simulink model "parent_model_2020a"  (R2020a)
settings: Solver=VariableStepAuto  StartTime=0.0  StopTime=10.0  RelTol=1e-3
libraries: sdl_lib x13, nesl_utility x9, autolibmappedmotor x4, autolibdatasheetbattery x1
settings Model: Creator=True  LastModifiedBy=True

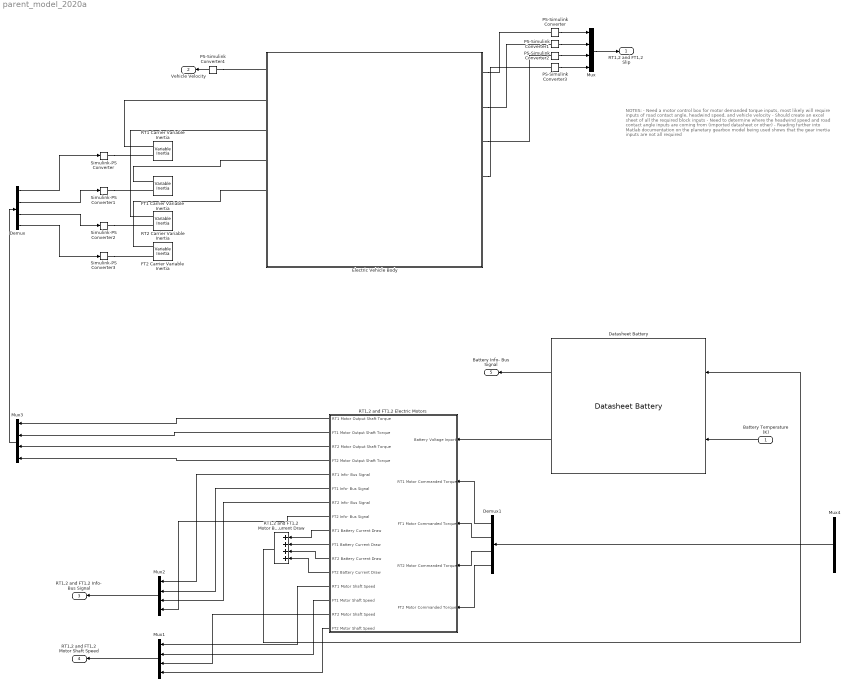
== system parent_model_2020a ==
  note: NOTES:
      | - Need a motor control box for motor demanded torque inputs, most likely will require inputs of road contact angle, headwind speed, and vehicle velocity
      |
      | - Should create an excel sheet of all the required block inputs
      |
      | - Need to determine where the headwind speed and road contact angle inputs are coming from (imported datasheet or other)
      |
      | - Reading further into Matlab documentation on the planetary gearbox model being used shows that the gear inertia inputs are not all required
  Battery Temperature (K) : Inport
  Datasheet Battery : autolibdatasheetbattery/Datasheet Battery  CapacityCtrl=Parameter  OutputVlt=Unfiltered  BattChargeMax=100  Em=[2.8 3.228 3.284 3.361 3.408 3.427 3.472 3.477 3.493 3.504 3.516 3.528 3.537 3.545 3.555 3.561 3.566 3.576 3.587 3.589 3.594 3.6 3.608 3.61 3.616 3.619 3.626 3.632 3.637 3.64 3.645 3.646 3.652 3.655 3.658 3.661 3.664 3.668 3.673 3.678 3.68 3.681 3.686 3.692 3.699 3.702 3.705 3.71 3.717 3.723 3.728 3.733 3.735 3.742 3.749 3.755 3.761 3.768 3.773 3.78 3.791 3.798 3.798 3.814 3.818 3.825 3.841 3.846 3.855 3.863 3.877 3.885 3.894 3.907 3.919 3.926 3.935 3.944 3.954 3.964 3.974 3.988 3.998 4.014 4.029 4.034 4.047 4.065 4.074 4.086 4.097 4.131 4.126 4.138 4.15 4.18 4.174 4.187 4.207 4.231 4.221]  CapLUTBp=[0 0.01 0.02 0.03 0.04 0.05 0.06 0.07 0.08 0.09 0.1 0.11 0.12 0.13 0.14 0.15 0.16 0.17 0.18 0.19 0.2 0.21 0.22 0.23 0.24 0.25 0.26 0.27 0.28 0.29 0.3 0.31 0.32 0.33 0.34 0.35 0.36 0.37 0.38 0.39 0.4 0.41 0.42 0.43 0.44 0.45 0.46 0.47 0.48 0.49 0.5 0.51 0.52 0.53 0.54 0.55 0.56 0.57 0.58 0.59 0.6 0.61 0.62 0.63 0.64 0.65 0.66 0.67 0.68 0.69 0.7 0.71 0.72 0.73 0.74 0.75 0.76 0.77 0.78 0.79 0.8 0.81 0.82 0.83 0.84 0.85 0.86 0.87 0.88 0.89 0.9 0.91 0.92 0.93 0.94 0.95 0.96 0.97 0.98 0.99 1]  RInt=[0.008846 0.009319 0.009027 0.00847 0.01032 0.01314;0.006389 0.006554 0.005553 0.005525 0.006043 0.007805;0.004364 0.004101 0.00406 0.003452 0.003846 0.004517;0.002031 0.002563 0.002532 0.00246 0.002716 0.003047;0.001443 0.001825 0.001795 0.001778 0.001924 0.002234;0.0005603 0.0007192 0.0006887 0.0007557 0.0007355 0.001014;0.001028 0.001338 0.001 0.001536 0.001546 0.002789]  BattTempBp=[243.1 253.1 263.1 273.1 283.1 298.1 313.1]  CapSOCBp=[0 0.2 0.4 0.6 0.8 1]  Ns=1  Np=1  BattCapInit=100  Tc=1/1000  Vinit=4.221  RefBlkName='autolibdatasheetbattery/Datasheet Battery'
      settings: SourceProductBaseCode=PW
  Demux : Demux
  Demux1 : Demux
  Electric Vehicle Body : Subsystem
      settings: PortSchema="{\"entries\":[{\"content\":{\"sides\":[{\"content\":{\"connectorIds\":[\"LConn1\",\"LConn2\",\"LConn3\",\"LConn4\",\"LConn5\",\"LConn6\",\"LConn7\"]},\"type\":\"ConnectorPlacement.EquallySpacedRectSide\",\"uuid\":\"0dd2967e-b693-4000-b07d-0da4332b2d76\"},{\"content\":{\"connectorIds\":[\"RConn1\",\"RConn2\",\"RConn3\",\"RConn4\",\"RConn5\",\"RConn6\"],\"side\":\"RIGHT\"},\"type\":\"ConnectorPlacement.EquallySpacedRectSide\",\"uuid\":\"63e3cb5e-c086-4dc9-bb10-408baad2e543\"},{\"content\":{\"connectorIds\":[\"LConn8\",\"LConn9\"],\"side\":\"TOP\"},\"type\":\"ConnectorPlacement.EquallySpacedRectSide\",\"uuid\":\"38187d83-6583-4cec-b53d-848b96f437cb\"}]},\"type\":\"ConnectorPlacement.EquallySpacedConnector\",\"uuid\":\"033be76d-f69f-4630-af0a-af49410de0d3\"}],\"packageUris\":[\"http://schema.mathworks.com/mf0/Connector/19700101\"],\"version\":\"1.0\"}"
  FT1 Carrier Variable Inertia : sdl_lib/Inertias & Loads/Variable Inertia  minimum_inertia=0.1 kg*m^2  L_specify=off  L_priority=High  L=0 m^2*kg/s  L_nominal_specify=off  L_nominal_unit=m^2*kg/s  L_nominal_value=1
      settings: SourceProductBaseCode=LD  InternalSimscapePortConfiguration="{\"Bottom\":[],\"Left\":[{\"id\":\"I\",\"label\":\"\",\"type\":\"input\"},{\"id\":\"A\",\"label\":\"\",\"type\":\"foundation.mechanical.rotational.rotational\"}],\"Right\":[],\"Top\":[]}"
  FT2 Carrier Variable Inertia : sdl_lib/Inertias & Loads/Variable Inertia  minimum_inertia=0.1 kg*m^2  L_specify=off  L_priority=High  L=0 m^2*kg/s  L_nominal_specify=off  L_nominal_unit=m^2*kg/s  L_nominal_value=1
      settings: SourceProductBaseCode=LD  InternalSimscapePortConfiguration="{\"Bottom\":[],\"Left\":[{\"id\":\"I\",\"label\":\"\",\"type\":\"input\"},{\"id\":\"A\",\"label\":\"\",\"type\":\"foundation.mechanical.rotational.rotational\"}],\"Right\":[],\"Top\":[]}"
  Mux{,1..4} (5 alike) : Mux
  PS-Simulink Converter{,1..4} (5 alike) : nesl_utility/PS-Simulink Converter  PhysicalDomain=network_engine_domain  SubClassName=ps_output  LeftPortType=input  RightPortType=output  PseudoPeriodic=off  Frequencies=[]  Unit=inherit  AffineConversion=off
  RT1 Carrier Variable Inertia : sdl_lib/Inertias & Loads/Variable Inertia  minimum_inertia=0.1 kg*m^2  L_specify=off  L_priority=High  L=0 m^2*kg/s  L_nominal_specify=off  L_nominal_unit=m^2*kg/s  L_nominal_value=1
      settings: SourceProductBaseCode=LD  InternalSimscapePortConfiguration="{\"Bottom\":[],\"Left\":[{\"id\":\"I\",\"label\":\"\",\"type\":\"input\"},{\"id\":\"A\",\"label\":\"\",\"type\":\"foundation.mechanical.rotational.rotational\"}],\"Right\":[],\"Top\":[]}"
  RT1,2 and FT1,2 Electric Motors : Subsystem
  RT1,2 and FT1,2 Motor Battery Current Draw : Sum  Inputs=++++
  RT2 Carrier Variable Inertia : sdl_lib/Inertias & Loads/Variable Inertia  minimum_inertia=0.1 kg*m^2  L_specify=off  L_priority=High  L=0 m^2*kg/s  L_nominal_specify=off  L_nominal_unit=m^2*kg/s  L_nominal_value=1
      settings: SourceProductBaseCode=LD  InternalSimscapePortConfiguration="{\"Bottom\":[],\"Left\":[{\"id\":\"I\",\"label\":\"\",\"type\":\"input\"},{\"id\":\"A\",\"label\":\"\",\"type\":\"foundation.mechanical.rotational.rotational\"}],\"Right\":[],\"Top\":[]}"
  Simulink-PS Converter{,1..3} (4 alike) : nesl_utility/Simulink-PS Converter  PhysicalDomain=network_engine_domain  SubClassName=ps_input  LeftPortType=input  RightPortType=output  PseudoPeriodic=off  Frequencies=[]  NoiseDistribution=none  NoiseParameters=[]  Unit=1  AffineConversion=off  FilteringAndDerivatives=provide  SimscapeFilterOrder=1  InputFilterTimeConstant=0.001  UdotUserProvided=0
  RT1,2 and FT1,2 Slip : Outport
  Vehicle Velocity : Outport  Port=2
  RT1,2 and FT1,2 Info- Bus Signal : Outport  Port=3
  RT1,2 and FT1,2 Motor Shaft Speed : Outport  Port=4
  Battery Info- Bus Signal : Outport  Port=5
  wires:
  Datasheet Battery/2 -> RT1,2 and FT1,2 Electric Motors/1(Battery Voltage Inport)
  RT1,2 and FT1,2 Electric Motors/9(RT1 Battery Current Draw) -> RT1,2 and FT1,2 Motor Battery Current Draw/1
  RT1,2 and FT1,2 Electric Motors/10(FT1 Battery Current Draw) -> RT1,2 and FT1,2 Motor Battery Current Draw/2
  RT1,2 and FT1,2 Electric Motors/11(RT2 Battery Current Draw) -> RT1,2 and FT1,2 Motor Battery Current Draw/3
  RT1,2 and FT1,2 Electric Motors/12(FT2 Battery Current Draw) -> RT1,2 and FT1,2 Motor Battery Current Draw/4
  RT1,2 and FT1,2 Motor Battery Current Draw/1 -> Datasheet Battery/1
  Battery Temperature (K)/1 -> Datasheet Battery/2
  PS-Simulink Converter/1 -> Mux/1
  PS-Simulink Converter1/1 -> Mux/2
  PS-Simulink Converter2/1 -> Mux/3
  PS-Simulink Converter3/1 -> Mux/4
  Mux/1 -> RT1,2 and FT1,2 Slip/1
  PS-Simulink Converter4/1 -> Vehicle Velocity/1
  RT1,2 and FT1,2 Electric Motors/5(RT1 Info- Bus Signal) -> Mux2/1
  RT1,2 and FT1,2 Electric Motors/6(FT1 Info- Bus Signal) -> Mux2/2
  RT1,2 and FT1,2 Electric Motors/7(RT2 Info- Bus Signal) -> Mux2/3
  RT1,2 and FT1,2 Electric Motors/8(FT2 Info- Bus Signal) -> Mux2/4
  RT1,2 and FT1,2 Electric Motors/13(RT1 Motor Shaft Speed) -> Mux1/1
  RT1,2 and FT1,2 Electric Motors/14(FT1 Motor Shaft Speed) -> Mux1/2
  RT1,2 and FT1,2 Electric Motors/15(RT2 Motor Shaft Speed) -> Mux1/3
  RT1,2 and FT1,2 Electric Motors/16(FT2 Motor Shaft Speed) -> Mux1/4
  Mux2/1 -> RT1,2 and FT1,2 Info- Bus Signal/1
  Mux1/1 -> RT1,2 and FT1,2 Motor Shaft Speed/1
  Datasheet Battery/1 -> Battery Info- Bus Signal/1
  Demux/1 -> Simulink-PS Converter/1
  Demux/4 -> Simulink-PS Converter3/1
  Demux/3 -> Simulink-PS Converter2/1
  Demux/2 -> Simulink-PS Converter1/1
  RT1,2 and FT1,2 Electric Motors/1(RT1 Motor Output Shaft Torque) -> Mux3/1
  RT1,2 and FT1,2 Electric Motors/2(FT1 Motor Output Shaft Torque) -> Mux3/2
  RT1,2 and FT1,2 Electric Motors/3(RT2 Motor Output Shaft Torque) -> Mux3/3
  RT1,2 and FT1,2 Electric Motors/4(FT2 Motor Output Shaft Torque) -> Mux3/4
  Mux3/1 -> Demux/1
  Demux1/1 -> RT1,2 and FT1,2 Electric Motors/2(RT1 Motor Commanded Torque)
  Demux1/2 -> RT1,2 and FT1,2 Electric Motors/3("FT1 Motor Commanded Torque ")
  Demux1/3 -> RT1,2 and FT1,2 Electric Motors/4(RT2 Motor Commanded Torque)
  Demux1/4 -> RT1,2 and FT1,2 Electric Motors/5(FT2 Motor Commanded Torque)
  Mux4/1 -> Demux1/1
  connections:
  Simulink-PS Converter1/RConn1 -- FT1 Carrier Variable Inertia/LConn1
  Simulink-PS Converter2/RConn1 -- RT2 Carrier Variable Inertia/LConn1
  Simulink-PS Converter/RConn1 -- RT1 Carrier Variable Inertia/LConn1
  Simulink-PS Converter3/RConn1 -- FT2 Carrier Variable Inertia/LConn1
  Electric Vehicle Body/RConn1 -- PS-Simulink Converter/LConn1
  Electric Vehicle Body/RConn2 -- PS-Simulink Converter1/LConn1
  PS-Simulink Converter4/LConn1 -- Electric Vehicle Body/LConn1
  Electric Vehicle Body/LConn2 -- RT1 Carrier Variable Inertia/LConn2
  Electric Vehicle Body/LConn3 -- RT2 Carrier Variable Inertia/LConn2
  Electric Vehicle Body/LConn4 -- FT1 Carrier Variable Inertia/LConn2
  Electric Vehicle Body/LConn5 -- FT2 Carrier Variable Inertia/LConn2
  Electric Vehicle Body/RConn3 -- PS-Simulink Converter2/LConn1
  Electric Vehicle Body/RConn4 -- PS-Simulink Converter3/LConn1

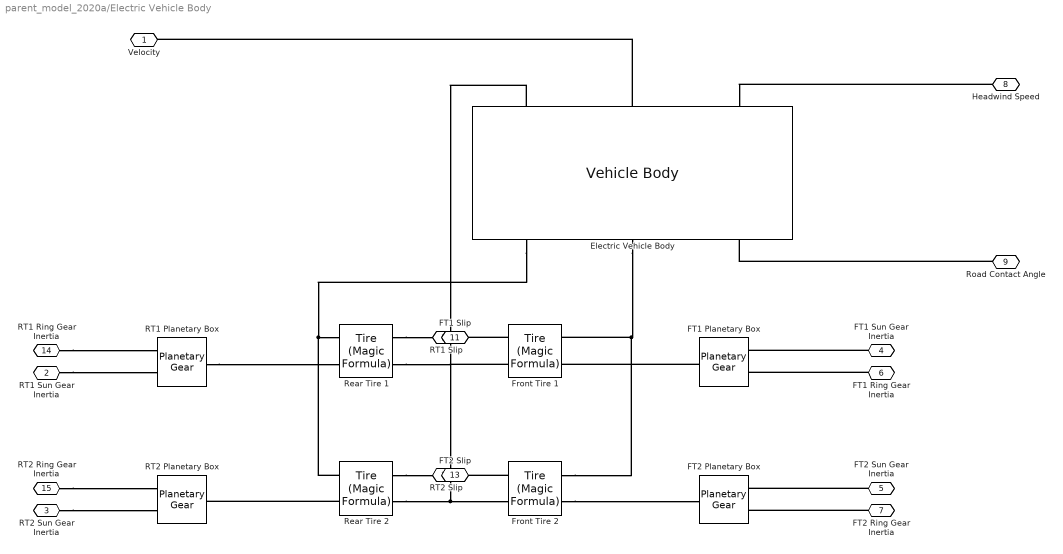
== system parent_model_2020a/Electric Vehicle Body ==
  Electric Vehicle Body : sdl_lib/Tires & Vehicles/Vehicle Body  mass=1200 kg  n_w=2  x_f=1.4 m  x_r=1.6 m  y_c=0.5 m  mass_var=simscape.enum.onoff.off  model_pitch=simscape.enum.onoff.on  inertia=4000 kg*m^2  suspension_model=sdl.enum.linearTLU.linear  k_f=1e4 N/m  b_f=1e4 N/(m/s)  k_r=1e4 N/m  b_r=1e4 N/(m/s)  k_f_TLU=[-2000, -1000, 0, 1000, 2000] N  x_f_TLU=[-.4, -.2, 0, .2, .4] m  b_f_TLU=[-200, -100, 0, 100, 200] N  v_f_TLU=[-4, -2, 0, 2, 4] m/s  k_r_TLU=[-2000, -1000, 0, 1000, 2000] N  x_r_TLU=[-.4, -.2, 0, .2, .4] m  b_r_TLU=[-200, -100, 0, 100, 200] N  v_r_TLU=[-4, -2, 0, 2, 4] m/s  interp_method=simscape.enum.interpolation.linear  extrap_method=simscape.enum.extrapolation.linear  model_hardstop=simscape.enum.onoff.off  upper_bound_f=.25 m  lower_bound_f=-.25 m  stop_k_f=1e6 N/m  stop_b_f=150 N/(m/s)  upper_bound_r=.25 m  lower_bound_r=-.25 m  stop_k_r=1e6 N/m  stop_b_r=150 N/(m/s)  initial_pitch=0 rad  initial_pitch_rate=0 rad/s  g=9.81 m/s^2  liftoff_warning=simscape.enum.onoff.off  area=3 m^2  Cd=0.4  rho=1.18 kg/m^3  v_specify=off  v_priority=High  v=0 m/s  v_nominal_specify=off  v_nominal_unit=m/s  v_nominal_value=1
  FT1 Planetary Box : sdl_lib/Gears/Planetary Gear  rs_ratio=2  friction_model=sdl.enum.gear_friction.none  mu_visc=[0, 0] N*m/(rad/s)  efficiency=[.96, .98]  temperature_TLU=[280, 300, 320] K  efficiency_sp_TLU=[.95, .9, .85]  efficiency_rp_TLU=[.95, .9, .85]  pwr_thr=[.001, .001] W  thermal_mass=50 J/K  T_init=300 K  model_inertia=simscape.enum.onoff.off  planet_inertia=0.001 kg*m^2
      settings: SourceProductBaseCode=LD
  FT2 Planetary Box : sdl_lib/Gears/Planetary Gear  rs_ratio=2  friction_model=sdl.enum.gear_friction.none  mu_visc=[0, 0] N*m/(rad/s)  efficiency=[.96, .98]  temperature_TLU=[280, 300, 320] K  efficiency_sp_TLU=[.95, .9, .85]  efficiency_rp_TLU=[.95, .9, .85]  pwr_thr=[.001, .001] W  thermal_mass=50 J/K  T_init=300 K  model_inertia=simscape.enum.onoff.off  planet_inertia=0.001 kg*m^2
      settings: SourceProductBaseCode=LD
  Front Tire 1 : sdl_lib/Tires & Vehicles/Tire (Magic Formula)  parameterization=sdl.enum.magic_tire_model.peak  F_z1=3000 N  F_x1=3500 N  kappa1=10  B_m=10  C_m=1.9  D_m=1  E_m=0.97  fz0=4000 N  p_Cx=1.685  p_Dx=[1.21, -.037]  p_Ex=[.344, .095, -.02, 0]  p_Kx=[21.51, -.163, .245]  p_Hx=[-.002, .002]  p_Vx=[0, 0]  v_tr_thr=0.1 m/s  r_e=0.3 m  model_compliance=0  stiffness=1e6 N/m  damping=1000 N/(m/s)  model_inertia=0  inertia=1 kg*m^2  initial_velocity=0 rad/s  model_resistance=0  resistance_model=1  coeff=0.015  p_tire=250e3 Pa  alpha=-0.003  beta=0.97  coeff_a=84e-4  coeff_b=6.2e-4 s/m  coeff_c=1.6e-4 s^2/m^2  v_thr=0.001 m/s
  Front Tire 2 : sdl_lib/Tires & Vehicles/Tire (Magic Formula)  parameterization=sdl.enum.magic_tire_model.peak  F_z1=3000 N  F_x1=3500 N  kappa1=10  B_m=10  C_m=1.9  D_m=1  E_m=0.97  fz0=4000 N  p_Cx=1.685  p_Dx=[1.21, -.037]  p_Ex=[.344, .095, -.02, 0]  p_Kx=[21.51, -.163, .245]  p_Hx=[-.002, .002]  p_Vx=[0, 0]  v_tr_thr=0.1 m/s  r_e=0.3 m  model_compliance=0  stiffness=1e6 N/m  damping=1000 N/(m/s)  model_inertia=0  inertia=1 kg*m^2  initial_velocity=0 rad/s  model_resistance=0  resistance_model=1  coeff=0.015  p_tire=250e3 Pa  alpha=-0.003  beta=0.97  coeff_a=84e-4  coeff_b=6.2e-4 s/m  coeff_c=1.6e-4 s^2/m^2  v_thr=0.001 m/s
  RT1 Planetary Box : sdl_lib/Gears/Planetary Gear  rs_ratio=2  friction_model=sdl.enum.gear_friction.none  mu_visc=[0, 0] N*m/(rad/s)  efficiency=[.96, .98]  temperature_TLU=[280, 300, 320] K  efficiency_sp_TLU=[.95, .9, .85]  efficiency_rp_TLU=[.95, .9, .85]  pwr_thr=[.001, .001] W  thermal_mass=50 J/K  T_init=300 K  model_inertia=simscape.enum.onoff.off  planet_inertia=0.001 kg*m^2
      settings: SourceProductBaseCode=LD
  RT2 Planetary Box : sdl_lib/Gears/Planetary Gear  rs_ratio=2  friction_model=sdl.enum.gear_friction.none  mu_visc=[0, 0] N*m/(rad/s)  efficiency=[.96, .98]  temperature_TLU=[280, 300, 320] K  efficiency_sp_TLU=[.95, .9, .85]  efficiency_rp_TLU=[.95, .9, .85]  pwr_thr=[.001, .001] W  thermal_mass=50 J/K  T_init=300 K  model_inertia=simscape.enum.onoff.off  planet_inertia=0.001 kg*m^2
      settings: SourceProductBaseCode=LD
  Rear Tire 1 : sdl_lib/Tires & Vehicles/Tire (Magic Formula)  parameterization=sdl.enum.magic_tire_model.peak  F_z1=3000 N  F_x1=3500 N  kappa1=10  B_m=10  C_m=1.9  D_m=1  E_m=0.97  fz0=4000 N  p_Cx=1.685  p_Dx=[1.21, -.037]  p_Ex=[.344, .095, -.02, 0]  p_Kx=[21.51, -.163, .245]  p_Hx=[-.002, .002]  p_Vx=[0, 0]  v_tr_thr=0.1 m/s  r_e=0.3 m  model_compliance=0  stiffness=1e6 N/m  damping=1000 N/(m/s)  model_inertia=0  inertia=1 kg*m^2  initial_velocity=0 rad/s  model_resistance=0  resistance_model=1  coeff=0.015  p_tire=250e3 Pa  alpha=-0.003  beta=0.97  coeff_a=84e-4  coeff_b=6.2e-4 s/m  coeff_c=1.6e-4 s^2/m^2  v_thr=0.001 m/s
  Rear Tire 2 : sdl_lib/Tires & Vehicles/Tire (Magic Formula)  parameterization=sdl.enum.magic_tire_model.peak  F_z1=3000 N  F_x1=3500 N  kappa1=10  B_m=10  C_m=1.9  D_m=1  E_m=0.97  fz0=4000 N  p_Cx=1.685  p_Dx=[1.21, -.037]  p_Ex=[.344, .095, -.02, 0]  p_Kx=[21.51, -.163, .245]  p_Hx=[-.002, .002]  p_Vx=[0, 0]  v_tr_thr=0.1 m/s  r_e=0.3 m  model_compliance=0  stiffness=1e6 N/m  damping=1000 N/(m/s)  model_inertia=0  inertia=1 kg*m^2  initial_velocity=0 rad/s  model_resistance=0  resistance_model=1  coeff=0.015  p_tire=250e3 Pa  alpha=-0.003  beta=0.97  coeff_a=84e-4  coeff_b=6.2e-4 s/m  coeff_c=1.6e-4 s^2/m^2  v_thr=0.001 m/s
  Velocity : PMIOPort  Side=Left
  RT1 Sun Gear Inertia : PMIOPort  Port=2  Side=Left
  RT2 Sun Gear Inertia : PMIOPort  Port=3  Side=Left
  FT1 Sun Gear Inertia : PMIOPort  Port=4  Side=Left
  FT2 Sun Gear Inertia : PMIOPort  Port=5  Side=Left
  FT1 Ring Gear Inertia : PMIOPort  Port=6  Side=Left
  FT2 Ring Gear Inertia : PMIOPort  Port=7  Side=Left
  Headwind Speed : PMIOPort  Port=8  Side=Left
  Road Contact Angle : PMIOPort  Port=9  Side=Left
  RT1 Slip : PMIOPort  Port=10  Side=Right
  FT1 Slip : PMIOPort  Port=11  Side=Right
  RT2 Slip : PMIOPort  Port=12  Side=Right
  FT2 Slip : PMIOPort  Port=13  Side=Right
  RT1 Ring Gear Inertia : PMIOPort  Port=14  Side=Right
  RT2 Ring Gear Inertia : PMIOPort  Port=15  Side=Right
  connections:
  Front Tire 2/LConn1 -- Front Tire 1/LConn1 -- Electric Vehicle Body/RConn2
  Rear Tire 2/LConn1 -- Rear Tire 1/LConn1 -- Electric Vehicle Body/RConn1
  Road Contact Angle/RConn1 -- Electric Vehicle Body/RConn3
  Rear Tire 2/RConn2 -- Front Tire 2/RConn2 -- Rear Tire 1/RConn2 -- Front Tire 1/RConn2 -- Electric Vehicle Body/LConn1
  Rear Tire 1/RConn1 -- RT1 Slip/RConn1
  Front Tire 1/RConn1 -- FT1 Slip/RConn1
  Headwind Speed/RConn1 -- Electric Vehicle Body/LConn3
  Front Tire 2/RConn1 -- FT2 Slip/RConn1
  Electric Vehicle Body/LConn2 -- Velocity/RConn1
  Rear Tire 2/RConn1 -- RT2 Slip/RConn1
  RT1 Ring Gear Inertia/RConn1 -- RT1 Planetary Box/RConn1
  RT1 Sun Gear Inertia/RConn1 -- RT1 Planetary Box/RConn2
  RT1 Planetary Box/LConn1 -- Rear Tire 1/LConn2
  RT2 Sun Gear Inertia/RConn1 -- RT2 Planetary Box/RConn2
  Rear Tire 2/LConn2 -- RT2 Planetary Box/LConn1
  RT2 Ring Gear Inertia/RConn1 -- RT2 Planetary Box/RConn1
  FT1 Sun Gear Inertia/RConn1 -- FT1 Planetary Box/RConn2
  FT1 Ring Gear Inertia/RConn1 -- FT1 Planetary Box/RConn1
  FT1 Planetary Box/LConn1 -- Front Tire 1/LConn2
  FT2 Sun Gear Inertia/RConn1 -- FT2 Planetary Box/RConn2
  FT2 Ring Gear Inertia/RConn1 -- FT2 Planetary Box/RConn1
  Front Tire 2/LConn2 -- FT2 Planetary Box/LConn1

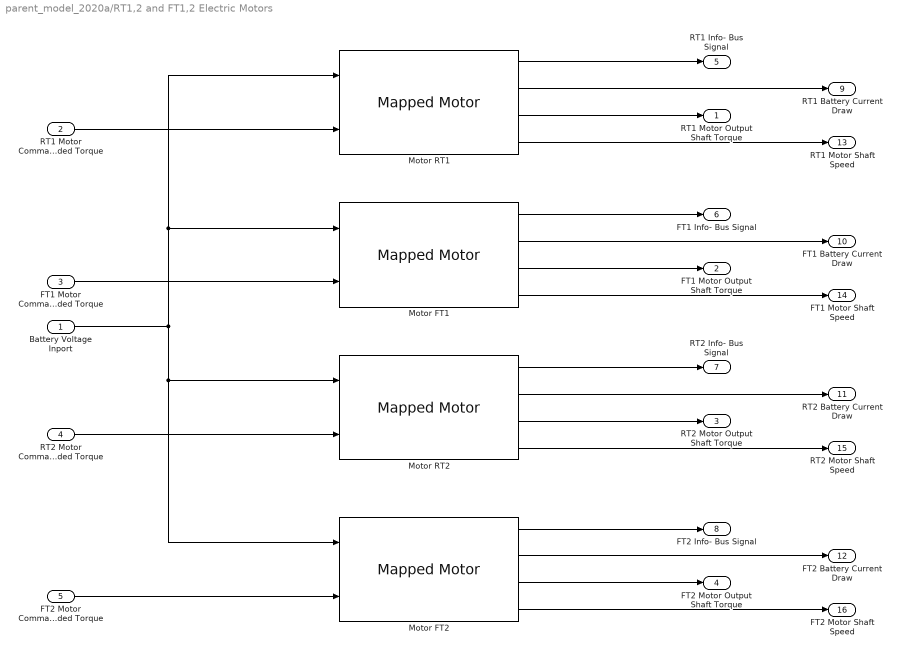
== system parent_model_2020a/RT1,2 and FT1,2 Electric Motors ==
  Battery Voltage Inport : Inport
  RT1 Motor Commanded Torque : Inport  Port=2
  "FT1 Motor Commanded Torque " : Inport  Port=3
  RT2 Motor Commanded Torque : Inport  Port=4
  FT2 Motor Commanded Torque : Inport  Port=5
  Motor FT1 : autolibmappedmotor/Mapped Motor  port_config=Torque  param_by=Tabulated torque-speed envelope  w_t=[ 0 375 750 800 ]  T_t=[0.09 0.08 0.07 0]  torque_max=.1  power_max=30  Tc=0.02  param_loss=Single efficiency measurement  eff=100  w_eff=375  T_eff=0.08  Piron=0  Pbase=0  w_eff_bp=[-8000 -4000 0 4000 8000]  T_eff_bp=[0 0.03 0.06 0.09]  Temp_eff_bp=[233.15 293.15 373.15]  losses_table=[1.49 1.67 2.21 3.10; 0.42 0.69 1.14 2.03; 0.06 0.24 0.78 1.68; 0.42 0.69 1.14 2.03; 1.49 1.67 2.21 3.10]  losses_table_3d=cat(3,[1.49 1.67 2.21 3.10; 0.42 0.69 1.14 2.03; 0.06 0.24 0.78 1.68; 0.42 0.69 1.14 2.03; 1.49 1.67 2.21 3.10],[1.49 1.67 2.21 3.10; 0.42 0.69 1.14 2.03; 0.06 0.24 0.78 1.68; 0.42 0.69 1.14 2.03; 1.49 1.67 2.21 3.10],[1.49 1.67 2.21 3.10; 0.42 0.69 1.14 2.03; 0.06 0.24 0.78 1.68; 0.42 0.69 1.14 2.03; 1.49 1.67 2.21 3.10])  efficiency_table=[95 95 95 95; 95 95 95 95; 95 95 95 95; 95 95 95 95; 95 95 95 95]  efficiency_table_3d=cat(3,[95 95 95 95; 95 95 95 95; 95 95 95 95; 95 95 95 95; 95 95 95 95],[95 95 95 95; 95 95 95 95; 95 95 95 95; 95 95 95 95; 95 95 95 95],[95 95 95 95; 95 95 95 95; 95 95 95 95; 95 95 95 95; 95 95 95 95])  J=5e-6  b=1e-5  omega_o=0  T_t_extended=[0 0.07 0.08 0.09 0.08 0.07 0]  w_t_extended=[-800 -750 -375 0 375 750 800]  KLossIron=0  KLossCopper=0  x_w_eff_vec=[-8000 -4000 0 4000 8000]  x_T_eff_vec=[-0.09 -0.06 -0.03 0 0.03 0.06 0.09]  x_tmp_eff_vec=[-0.09 -0.06 -0.03 0 0.03 0.06 0.09]  x_losses_mat=[3.1 2.21 1.67 1.49 1.67 2.21 3.1;2.03 1.14 0.69 0.42 0.69 1.14 2.03;1.68 0.78 0.24 0.06 0.24 0.78 1.68;2.03 1.14 0.69 0.42 0.69 1.14 2.03;3.1 2.21 1.67 1.49 1.67 2.21 3.1]  x_losses_mat_3d=[37.8947368421052 25.2631578947368 12.6315789473684 0 12 24 36;18.9473684210526 12.6315789473684 6.3157894736842 0 5.99999999999999 12 18;0 0 0 0 0 0 0;18 12 5.99999999999999 0 6.3157894736842 12.6315789473684 18.9473684210526;36 24 12 0 12.6315789473684 25.2631578947368 37.8947368421052]  CalLossMapData={}  CalLossWithTempMapData={}  aMode=1  RefBlkName='autolibmappedmotor/Mapped Motor'
      settings: SourceProductBaseCode=PW,MT,UV,VE,VP
  Motor FT2 : autolibmappedmotor/Mapped Motor  port_config=Torque  param_by=Tabulated torque-speed envelope  w_t=[ 0 375 750 800 ]  T_t=[0.09 0.08 0.07 0]  torque_max=.1  power_max=30  Tc=0.02  param_loss=Single efficiency measurement  eff=100  w_eff=375  T_eff=0.08  Piron=0  Pbase=0  w_eff_bp=[-8000 -4000 0 4000 8000]  T_eff_bp=[0 0.03 0.06 0.09]  Temp_eff_bp=[233.15 293.15 373.15]  losses_table=[1.49 1.67 2.21 3.10; 0.42 0.69 1.14 2.03; 0.06 0.24 0.78 1.68; 0.42 0.69 1.14 2.03; 1.49 1.67 2.21 3.10]  losses_table_3d=cat(3,[1.49 1.67 2.21 3.10; 0.42 0.69 1.14 2.03; 0.06 0.24 0.78 1.68; 0.42 0.69 1.14 2.03; 1.49 1.67 2.21 3.10],[1.49 1.67 2.21 3.10; 0.42 0.69 1.14 2.03; 0.06 0.24 0.78 1.68; 0.42 0.69 1.14 2.03; 1.49 1.67 2.21 3.10],[1.49 1.67 2.21 3.10; 0.42 0.69 1.14 2.03; 0.06 0.24 0.78 1.68; 0.42 0.69 1.14 2.03; 1.49 1.67 2.21 3.10])  efficiency_table=[95 95 95 95; 95 95 95 95; 95 95 95 95; 95 95 95 95; 95 95 95 95]  efficiency_table_3d=cat(3,[95 95 95 95; 95 95 95 95; 95 95 95 95; 95 95 95 95; 95 95 95 95],[95 95 95 95; 95 95 95 95; 95 95 95 95; 95 95 95 95; 95 95 95 95],[95 95 95 95; 95 95 95 95; 95 95 95 95; 95 95 95 95; 95 95 95 95])  J=5e-6  b=1e-5  omega_o=0  T_t_extended=[0 0.07 0.08 0.09 0.08 0.07 0]  w_t_extended=[-800 -750 -375 0 375 750 800]  KLossIron=0  KLossCopper=0  x_w_eff_vec=[-8000 -4000 0 4000 8000]  x_T_eff_vec=[-0.09 -0.06 -0.03 0 0.03 0.06 0.09]  x_tmp_eff_vec=[-0.09 -0.06 -0.03 0 0.03 0.06 0.09]  x_losses_mat=[3.1 2.21 1.67 1.49 1.67 2.21 3.1;2.03 1.14 0.69 0.42 0.69 1.14 2.03;1.68 0.78 0.24 0.06 0.24 0.78 1.68;2.03 1.14 0.69 0.42 0.69 1.14 2.03;3.1 2.21 1.67 1.49 1.67 2.21 3.1]  x_losses_mat_3d=[37.8947368421052 25.2631578947368 12.6315789473684 0 12 24 36;18.9473684210526 12.6315789473684 6.3157894736842 0 5.99999999999999 12 18;0 0 0 0 0 0 0;18 12 5.99999999999999 0 6.3157894736842 12.6315789473684 18.9473684210526;36 24 12 0 12.6315789473684 25.2631578947368 37.8947368421052]  CalLossMapData={}  CalLossWithTempMapData={}  aMode=1  RefBlkName='autolibmappedmotor/Mapped Motor'
      settings: SourceProductBaseCode=PW,MT,UV,VE,VP
  Motor RT1 : autolibmappedmotor/Mapped Motor  port_config=Torque  param_by=Tabulated torque-speed envelope  w_t=[ 0 375 750 800 ]  T_t=[0.09 0.08 0.07 0]  torque_max=.1  power_max=30  Tc=0.02  param_loss=Single efficiency measurement  eff=100  w_eff=375  T_eff=0.08  Piron=0  Pbase=0  w_eff_bp=[-8000 -4000 0 4000 8000]  T_eff_bp=[0 0.03 0.06 0.09]  Temp_eff_bp=[233.15 293.15 373.15]  losses_table=[1.49 1.67 2.21 3.10; 0.42 0.69 1.14 2.03; 0.06 0.24 0.78 1.68; 0.42 0.69 1.14 2.03; 1.49 1.67 2.21 3.10]  losses_table_3d=cat(3,[1.49 1.67 2.21 3.10; 0.42 0.69 1.14 2.03; 0.06 0.24 0.78 1.68; 0.42 0.69 1.14 2.03; 1.49 1.67 2.21 3.10],[1.49 1.67 2.21 3.10; 0.42 0.69 1.14 2.03; 0.06 0.24 0.78 1.68; 0.42 0.69 1.14 2.03; 1.49 1.67 2.21 3.10],[1.49 1.67 2.21 3.10; 0.42 0.69 1.14 2.03; 0.06 0.24 0.78 1.68; 0.42 0.69 1.14 2.03; 1.49 1.67 2.21 3.10])  efficiency_table=[95 95 95 95; 95 95 95 95; 95 95 95 95; 95 95 95 95; 95 95 95 95]  efficiency_table_3d=cat(3,[95 95 95 95; 95 95 95 95; 95 95 95 95; 95 95 95 95; 95 95 95 95],[95 95 95 95; 95 95 95 95; 95 95 95 95; 95 95 95 95; 95 95 95 95],[95 95 95 95; 95 95 95 95; 95 95 95 95; 95 95 95 95; 95 95 95 95])  J=5e-6  b=1e-5  omega_o=0  T_t_extended=[0 0.07 0.08 0.09 0.08 0.07 0]  w_t_extended=[-800 -750 -375 0 375 750 800]  KLossIron=0  KLossCopper=0  x_w_eff_vec=[-8000 -4000 0 4000 8000]  x_T_eff_vec=[-0.09 -0.06 -0.03 0 0.03 0.06 0.09]  x_tmp_eff_vec=[-0.09 -0.06 -0.03 0 0.03 0.06 0.09]  x_losses_mat=[3.1 2.21 1.67 1.49 1.67 2.21 3.1;2.03 1.14 0.69 0.42 0.69 1.14 2.03;1.68 0.78 0.24 0.06 0.24 0.78 1.68;2.03 1.14 0.69 0.42 0.69 1.14 2.03;3.1 2.21 1.67 1.49 1.67 2.21 3.1]  x_losses_mat_3d=[37.8947368421052 25.2631578947368 12.6315789473684 0 12 24 36;18.9473684210526 12.6315789473684 6.3157894736842 0 5.99999999999999 12 18;0 0 0 0 0 0 0;18 12 5.99999999999999 0 6.3157894736842 12.6315789473684 18.9473684210526;36 24 12 0 12.6315789473684 25.2631578947368 37.8947368421052]  CalLossMapData={}  CalLossWithTempMapData={}  aMode=1  RefBlkName='autolibmappedmotor/Mapped Motor'
      settings: SourceProductBaseCode=PW,MT,UV,VE,VP
  Motor RT2 : autolibmappedmotor/Mapped Motor  port_config=Torque  param_by=Tabulated torque-speed envelope  w_t=[ 0 375 750 800 ]  T_t=[0.09 0.08 0.07 0]  torque_max=.1  power_max=30  Tc=0.02  param_loss=Single efficiency measurement  eff=100  w_eff=375  T_eff=0.08  Piron=0  Pbase=0  w_eff_bp=[-8000 -4000 0 4000 8000]  T_eff_bp=[0 0.03 0.06 0.09]  Temp_eff_bp=[233.15 293.15 373.15]  losses_table=[1.49 1.67 2.21 3.10; 0.42 0.69 1.14 2.03; 0.06 0.24 0.78 1.68; 0.42 0.69 1.14 2.03; 1.49 1.67 2.21 3.10]  losses_table_3d=cat(3,[1.49 1.67 2.21 3.10; 0.42 0.69 1.14 2.03; 0.06 0.24 0.78 1.68; 0.42 0.69 1.14 2.03; 1.49 1.67 2.21 3.10],[1.49 1.67 2.21 3.10; 0.42 0.69 1.14 2.03; 0.06 0.24 0.78 1.68; 0.42 0.69 1.14 2.03; 1.49 1.67 2.21 3.10],[1.49 1.67 2.21 3.10; 0.42 0.69 1.14 2.03; 0.06 0.24 0.78 1.68; 0.42 0.69 1.14 2.03; 1.49 1.67 2.21 3.10])  efficiency_table=[95 95 95 95; 95 95 95 95; 95 95 95 95; 95 95 95 95; 95 95 95 95]  efficiency_table_3d=cat(3,[95 95 95 95; 95 95 95 95; 95 95 95 95; 95 95 95 95; 95 95 95 95],[95 95 95 95; 95 95 95 95; 95 95 95 95; 95 95 95 95; 95 95 95 95],[95 95 95 95; 95 95 95 95; 95 95 95 95; 95 95 95 95; 95 95 95 95])  J=5e-6  b=1e-5  omega_o=0  T_t_extended=[0 0.07 0.08 0.09 0.08 0.07 0]  w_t_extended=[-800 -750 -375 0 375 750 800]  KLossIron=0  KLossCopper=0  x_w_eff_vec=[-8000 -4000 0 4000 8000]  x_T_eff_vec=[-0.09 -0.06 -0.03 0 0.03 0.06 0.09]  x_tmp_eff_vec=[-0.09 -0.06 -0.03 0 0.03 0.06 0.09]  x_losses_mat=[3.1 2.21 1.67 1.49 1.67 2.21 3.1;2.03 1.14 0.69 0.42 0.69 1.14 2.03;1.68 0.78 0.24 0.06 0.24 0.78 1.68;2.03 1.14 0.69 0.42 0.69 1.14 2.03;3.1 2.21 1.67 1.49 1.67 2.21 3.1]  x_losses_mat_3d=[37.8947368421052 25.2631578947368 12.6315789473684 0 12 24 36;18.9473684210526 12.6315789473684 6.3157894736842 0 5.99999999999999 12 18;0 0 0 0 0 0 0;18 12 5.99999999999999 0 6.3157894736842 12.6315789473684 18.9473684210526;36 24 12 0 12.6315789473684 25.2631578947368 37.8947368421052]  CalLossMapData={}  CalLossWithTempMapData={}  aMode=1  RefBlkName='autolibmappedmotor/Mapped Motor'
      settings: SourceProductBaseCode=PW,MT,UV,VE,VP
  RT1 Motor Output Shaft Torque : Outport
  FT1 Motor Output Shaft Torque : Outport  Port=2
  RT2 Motor Output Shaft Torque : Outport  Port=3
  FT2 Motor Output Shaft Torque : Outport  Port=4
  RT1 Info- Bus Signal : Outport  Port=5
  FT1 Info- Bus Signal : Outport  Port=6
  RT2 Info- Bus Signal : Outport  Port=7
  FT2 Info- Bus Signal : Outport  Port=8
  RT1 Battery Current Draw : Outport  Port=9
  FT1 Battery Current Draw : Outport  Port=10
  RT2 Battery Current Draw : Outport  Port=11
  FT2 Battery Current Draw : Outport  Port=12
  RT1 Motor Shaft Speed : Outport  Port=13
  FT1 Motor Shaft Speed : Outport  Port=14
  RT2 Motor Shaft Speed : Outport  Port=15
  FT2 Motor Shaft Speed : Outport  Port=16
  wires:
  Motor FT2/3 -> FT2 Motor Output Shaft Torque/1
  Battery Voltage Inport/1 -> Motor RT2/1, Motor FT2/1, Motor FT1/1, Motor RT1/1
  Motor RT1/1 -> RT1 Info- Bus Signal/1
  RT1 Motor Commanded Torque/1 -> Motor RT1/2
  "FT1 Motor Commanded Torque "/1 -> Motor FT1/2
  Motor RT2/1 -> RT2 Info- Bus Signal/1
  Motor FT1/1 -> FT1 Info- Bus Signal/1
  Motor FT2/1 -> FT2 Info- Bus Signal/1
  Motor FT1/4 -> FT1 Motor Shaft Speed/1
  FT2 Motor Commanded Torque/1 -> Motor FT2/2
  Motor RT2/4 -> RT2 Motor Shaft Speed/1
  Motor RT2/2 -> RT2 Battery Current Draw/1
  Motor FT2/4 -> FT2 Motor Shaft Speed/1
  Motor FT2/2 -> FT2 Battery Current Draw/1
  Motor RT1/3 -> RT1 Motor Output Shaft Torque/1
  RT2 Motor Commanded Torque/1 -> Motor RT2/2
  Motor RT1/4 -> RT1 Motor Shaft Speed/1
  Motor FT1/3 -> FT1 Motor Output Shaft Torque/1
  Motor RT2/3 -> RT2 Motor Output Shaft Torque/1
  Motor RT1/2 -> RT1 Battery Current Draw/1
  Motor FT1/2 -> FT1 Battery Current Draw/1
